simulink model "starmac_system_embedded_test"  (Simulink 7.1)
settings: Solver=ode23  StartTime=0.0  StopTime=80  FixedStep=.001  MaxStep=.01  RelTol=1e-4
libraries: aero_sim_lib x7, control_design_lib x6, simulink x4
(part 1 of 2)
settings Model: Creator=Administrator  LastModifiedBy=jporter

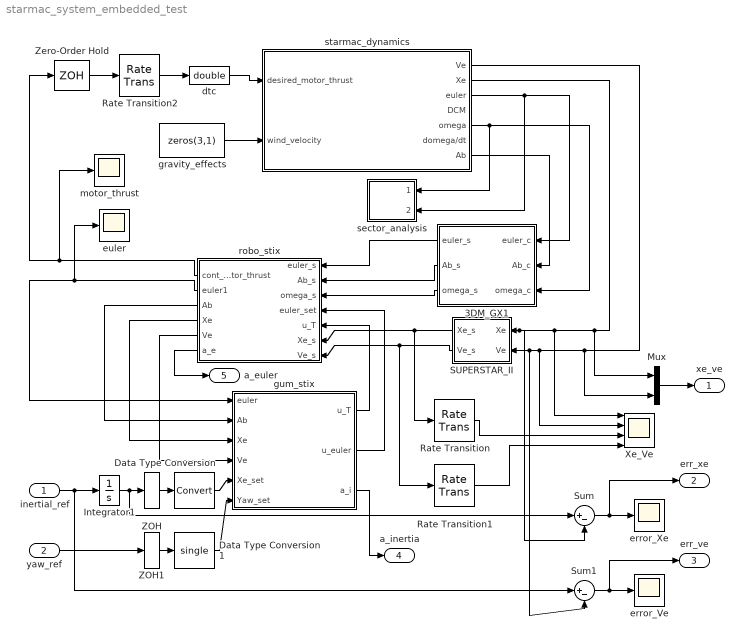
== system starmac_system_embedded_test ==
  inertial_ref : Inport  OutDataType=sfix(16)  OutScaling=2^0
  yaw_ref : Inport  Port=2  OutDataType=sfix(16)  OutScaling=2^0
  3DM_GX1 : Subsystem  Orientation=left  mask{a_g_s=7000, g_max=5, g_g_s=8500, omega_max=300, Ts=.02}
      mask prompts: a_g_s "AccelGainScale:"; g_max "Max G (1 G = 9.81 m/s^2):"; g_g_s "GyroGainScale:"; omega_max "Mav Angular Velocity (deg/sec):"; Ts "Sample Rate (seconds):"
  Data Type Conversion : DataTypeConversion  OutDataType=sfix(16)  OutScaling=2^0
  Data Type Conversion1 : DataTypeConversion  OutDataTypeMode=single  OutDataType=sfix(16)  OutScaling=2^0  OutDataTypeStr=single
  Integrator1 : Integrator
  Mux : Mux  Inputs=2
  Rate Transition : RateTransition
  Rate Transition1 : RateTransition
  Rate Transition2 : RateTransition
  SUPERSTAR_II : Subsystem  Orientation=left  mask{Ts=.02}
      mask prompts: Ts "Sample Rate (seconds):"
  Sum : Sum  Inputs=|+-  OutDataType=sfix(16)  OutScaling=2^0
  Sum1 : Sum  Inputs=|+-  OutDataType=sfix(16)  OutScaling=2^0
  Xe_Ve : Scope  NumInputPorts=4
      settings: YMin=-15~-6~-15~-6  YMax=15~5~15~5  Decimation=20
  ZOH : ZeroOrderHold  SampleTime=.02
  ZOH1 : ZeroOrderHold  SampleTime=.02
  Zero-Order Hold : ZeroOrderHold  SampleTime=.02
  dtc : DataTypeConversion  OutDataTypeMode=double  OutDataType=sfix(16)  OutScaling=2^0  OutDataTypeStr=double
  error_Ve : Scope
      settings: YMin=-4  SaveName=ScopeData14  Decimation=10
  error_Xe : Scope
      settings: YMin=-4  SaveName=ScopeData4  Decimation=10
  euler : Scope
      settings: TimeRange=60  YMin=-0.05  YMax=0.009999999999999995
  gravity_effects : Constant  Value=zeros(3,1)  OutDataTypeMode=double  OutDataType=sfix(16)  OutScaling=2^0  OutDataTypeStr=double
  gum_stix : Subsystem
  motor_thrust : Scope
      settings: YMin=2.5  YMax=10  SaveName=ScopeData3
  robo_stix : Subsystem  Orientation=left
  sector_analysis : Subsystem  Orientation=left
  starmac_dynamics : Subsystem  AncestorBlock=aero_sim_lib/starmac_dynamics  mask{M=1.8263, tau_motor=0.1, b=0.1, select_sub=Select Subsystem}
      mask prompts: M "UAV Mass (kg) [M]:"; tau_motor "Motor Time constant (s)[tau_motor]:"; b "Viscus Drag Coef. (N-s/m)[b]:"; select_sub "Select a model Subsystem:"
      mask StyleString: edit,edit,edit,popup(Select Subsystem|M:starmac_motor_dynamics|B:starmac_blade_flapping_effects|6:6DOF_Euler_Angles)
      mask CallbackString:
      | |||gcb_d=gcb;
      | mask_str = get_param(gcb_d, 'MaskValues');
      | if strcmp(mask_str{4}(1),'M')
      |     open_system([gcb_d '/starmac_motor_dynamics'],'mask');
      | elseif strcmp(mask_str{4}(1),'B')
      |     open_system([gcb_d '/starmac_blade_flapping_effects'],'mask');
      | elseif strcmp(mask_str{4}(1),'6')
      |     open_system([gcb_d '/6DOF_Euler_Angles'],'mask');
      | else
      |     return
      | end
      | set_param(gcb_d,'select_sub','Select Subsystem');
  xe_ve : Outport
  err_xe : Outport  Port=2
  err_ve : Outport  Port=3
  a_inertia : Outport  Port=4
  a_euler : Outport  Port=5
  wires:
  robo_stix/1(cont_motor_thrust) -> Zero-Order Hold/1, motor_thrust/1
  starmac_dynamics/3(euler) -> 3DM_GX1/1(euler_c), sector_analysis/2(out(eta))
  starmac_dynamics/7(Ab) -> 3DM_GX1/2(Ab_c)
  3DM_GX1/1(euler_s) -> robo_stix/1(euler_s)
  3DM_GX1/2(Ab_s) -> robo_stix/2(Ab_s)
  3DM_GX1/3(omega_s) -> robo_stix/3(omega_s)
  robo_stix/2(euler1) -> euler/1, gum_stix/1(euler)
  SUPERSTAR_II/1(Xe_s) -> Rate Transition/1, robo_stix/6(Xe_s)
  SUPERSTAR_II/2(Ve_s) -> Rate Transition1/1, robo_stix/7(Ve_s)
  starmac_dynamics/2(Xe) -> Xe_Ve/1, SUPERSTAR_II/1(Xe), Sum/2, Mux/1
  starmac_dynamics/1(Ve) -> Xe_Ve/2, SUPERSTAR_II/2(Ve), Sum1/2, Mux/2
  inertial_ref/1 -> Integrator1/1, Sum1/1
  gravity_effects/1 -> starmac_dynamics/2(wind_velocity)
  Sum/1 -> error_Xe/1, err_xe/1
  Rate Transition/1 -> Xe_Ve/3
  Rate Transition1/1 -> Xe_Ve/4
  gum_stix/1(u_T) -> robo_stix/5(u_T)
  gum_stix/2(u_euler) -> robo_stix/4(euler_set)
  Data Type Conversion/1 -> gum_stix/5(Xe_set)
  dtc/1 -> starmac_dynamics/1(desired_motor_thrust)
  starmac_dynamics/5(omega) -> 3DM_GX1/3(omega_c), sector_analysis/1(in(omega))
  Zero-Order Hold/1 -> Rate Transition2/1
  Rate Transition2/1 -> dtc/1
  robo_stix/3(Ab) -> gum_stix/2(Ab)
  robo_stix/4(Xe) -> gum_stix/3(Xe)
  robo_stix/5(Ve) -> gum_stix/4(Ve)
  Integrator1/1 -> ZOH/1, Sum/1
  ZOH/1 -> Data Type Conversion/1
  ZOH1/1 -> Data Type Conversion1/1
  yaw_ref/1 -> ZOH1/1
  Data Type Conversion1/1 -> gum_stix/6(Yaw_set)
  Mux/1 -> xe_ve/1
  Sum1/1 -> error_Ve/1, err_ve/1
  gum_stix/3(a_i) -> a_inertia/1
  robo_stix/6(a_e) -> a_euler/1

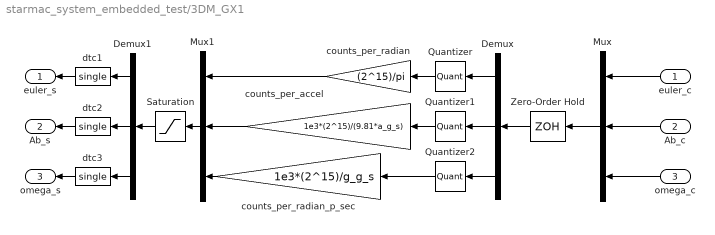
== system starmac_system_embedded_test/3DM_GX1 ==
  euler_c : Inport  Orientation=left
  Ab_c : Inport  Orientation=left  Port=2
  omega_c : Inport  Orientation=left  Port=3
  Demux : Demux  Orientation=left  Outputs=[3 3 3]
  Demux1 : Demux  Orientation=left  Outputs=[3 3 3]
  Mux : Mux  Orientation=left  Inputs=[3 3 3]
  Mux1 : Mux  Orientation=left  Inputs=3
  Quantizer : Quantizer  Orientation=left  QuantizationInterval=pi/(2^15)*ones(3,1)
  Quantizer1 : Quantizer  Orientation=left  QuantizationInterval=g_max*9.81/(2^15)*ones(3,1)
  Quantizer2 : Quantizer  Orientation=left  QuantizationInterval=(pi*omega_max/180)/(2^15)*ones(3,1)
  Saturation : Saturate  Orientation=left  UpperLimit=((2^15)-1)*ones(3*3,1)  LowerLimit=-(2^15)*ones(3*3,1)  OutDataType=sfix(16)  OutScaling=2^0
  Zero-Order Hold : ZeroOrderHold  Orientation=left  SampleTime=Ts
  counts_per_accel : Gain  Orientation=left  Gain=1e3*(2^15)/(9.81*a_g_s)  ParameterDataType=sfix(16)  ParameterScaling=2^0  OutDataType=sfix(16)  OutScaling=2^0
  counts_per_radian : Gain  Orientation=left  Gain=(2^15)/pi  ParameterDataType=sfix(16)  ParameterScaling=2^0  OutDataType=sfix(16)  OutScaling=2^0
  counts_per_radian_p_sec : Gain  Orientation=left  Gain=1e3*(2^15)/g_g_s  ParameterDataType=sfix(16)  ParameterScaling=2^0  OutDataType=sfix(16)  OutScaling=2^0
  dtc1 : DataTypeConversion  Orientation=left  OutDataTypeMode=single  OutDataType=sfix(16)  OutScaling=2^0  OutDataTypeStr=single
  dtc2 : DataTypeConversion  Orientation=left  OutDataTypeMode=single  OutDataType=sfix(16)  OutScaling=2^0  OutDataTypeStr=single
  dtc3 : DataTypeConversion  Orientation=left  OutDataTypeMode=single  OutDataType=sfix(16)  OutScaling=2^0  OutDataTypeStr=single
  euler_s : Outport  Orientation=left
  Ab_s : Outport  Orientation=left  Port=2
  omega_s : Outport  Orientation=left  Port=3
  wires:
  Mux/1 -> Zero-Order Hold/1
  euler_c/1 -> Mux/1
  Ab_c/1 -> Mux/2
  omega_c/1 -> Mux/3
  Zero-Order Hold/1 -> Demux/1
  Demux/1 -> Quantizer/1
  Demux/2 -> Quantizer1/1
  Quantizer/1 -> counts_per_radian/1
  Quantizer1/1 -> counts_per_accel/1
  counts_per_accel/1 -> Mux1/2
  counts_per_radian/1 -> Mux1/1
  Demux/3 -> Quantizer2/1
  counts_per_radian_p_sec/1 -> Mux1/3
  Quantizer2/1 -> counts_per_radian_p_sec/1
  Mux1/1 -> Saturation/1
  Saturation/1 -> Demux1/1
  Demux1/1 -> dtc1/1
  Demux1/2 -> dtc2/1
  Demux1/3 -> dtc3/1
  dtc1/1 -> euler_s/1
  dtc2/1 -> Ab_s/1
  dtc3/1 -> omega_s/1

== system starmac_system_embedded_test/SUPERSTAR_II ==
  Xe : Inport  Orientation=left
  Ve : Inport  Orientation=left  Port=2
  Demux : Demux  Orientation=left  Outputs=[3 3]
  Mux : Mux  Orientation=left  Inputs=[3 3]
  Rate Transition : RateTransition  Orientation=left
  ZOH : ZeroOrderHold  Orientation=left  SampleTime=Ts
  dtc1 : DataTypeConversion  Orientation=left  OutDataTypeMode=single  OutDataType=sfix(16)  OutScaling=2^0  OutDataTypeStr=single
  dtc2 : DataTypeConversion  Orientation=left  OutDataTypeMode=single  OutDataType=sfix(16)  OutScaling=2^0  OutDataTypeStr=single
  Xe_s : Outport  Orientation=left
  Ve_s : Outport  Orientation=left  Port=2
  wires:
  ZOH/1 -> Rate Transition/1
  Ve/1 -> Mux/2
  Xe/1 -> Mux/1
  Mux/1 -> ZOH/1
  Demux/1 -> dtc1/1
  Demux/2 -> dtc2/1
  dtc1/1 -> Xe_s/1
  dtc2/1 -> Ve_s/1
  Rate Transition/1 -> Demux/1

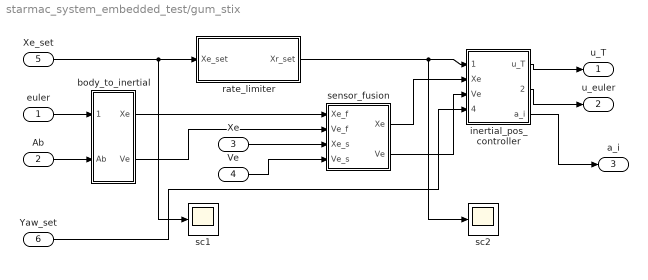
== system starmac_system_embedded_test/gum_stix ==
  euler : Inport  PortDimensions=[3]  DataType=single  OutDataTypeStr=single
  Ab : Inport  Port=2  PortDimensions=[3]  DataType=single  OutDataTypeStr=single
  Xe : Inport  Port=3  PortDimensions=[3]  DataType=single  OutDataTypeStr=single
  Ve : Inport  Port=4  PortDimensions=[3]  DataType=single  OutDataTypeStr=single
  Xe_set : Inport  Port=5  PortDimensions=[3]  DataType=single  OutDataTypeStr=single
  Yaw_set : Inport  Port=6  PortDimensions=[1]  DataType=single  OutDataTypeStr=single
  body_to_inertial : Subsystem
  inertial_pos_controller : Subsystem
  rate_limiter : Subsystem  mask{wn=2*pi, zeta=0.9, Vmax=2, Tsamp=0.02}
      mask prompts: wn "omega_n"; Vmax "Max velocity"; Tsamp "Sample time"
      mask init:
      | Fsys = tf([wn^2],[1,2*zeta*wn,wn^2]);
      | Fd = c2d( Fsys, Tsamp, 'zoh' );
      | FS = ss( Fd );
      | Add = FS.a;
      | Bdd = FS.b;
      | Cdd = FS.c;
      | Ddd = FS.d;
      | %Add = blkdiag(FS.a, FS.a, FS.a );
      | %Bdd = blkdiag(FS.b, FS.b, FS.b );
      | %Cdd = blkdiag(FS.c, FS.c, FS.c );
      | %Ddd = blkdiag(FS.d, FS.d, FS.d );
      | %Sdd = ss( Add, Bdd, Cdd, Ddd, Tsamp );
  sc1 : Scope
      settings: YMin=-7.5  YMax=22.5  SaveName=ScopeData8  Decimation=10
  sc2 : Scope
      settings: YMin=-2  YMax=2  SaveName=ScopeData9  Decimation=10
  sensor_fusion : Subsystem
  u_T : Outport  PortDimensions=[1]  DataType=single  OutDataTypeStr=single
  u_euler : Outport  Port=2  PortDimensions=[3]  DataType=single  OutDataTypeStr=single
  a_i : Outport  Port=3
  wires:
  Xe_set/1 -> rate_limiter/1(Xe_set), sc1/1
  inertial_pos_controller/1(u_T) -> u_T/1
  inertial_pos_controller/2(u_euler) -> u_euler/1
  euler/1 -> body_to_inertial/1(euler)
  Ab/1 -> body_to_inertial/2(Ab)
  sensor_fusion/1(Xe) -> inertial_pos_controller/2(Xe)
  sensor_fusion/2(Ve) -> inertial_pos_controller/3(Ve)
  body_to_inertial/1(Xe) -> sensor_fusion/1(Xe_f)
  body_to_inertial/2(Ve) -> sensor_fusion/2(Ve_f)
  Xe/1 -> sensor_fusion/3(Xe_s)
  Ve/1 -> sensor_fusion/4(Ve_s)
  rate_limiter/1(Xr_set) -> inertial_pos_controller/1(Xe_set), sc2/1
  Yaw_set/1 -> inertial_pos_controller/4(Yaw_set)
  inertial_pos_controller/3(a_i) -> a_i/1

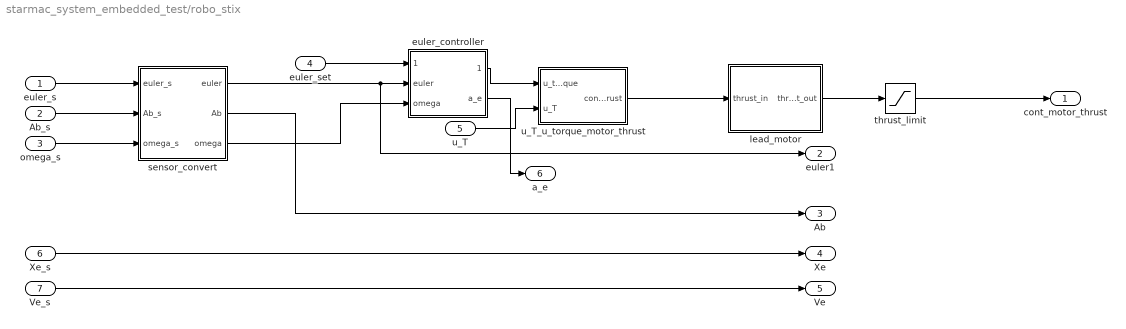
== system starmac_system_embedded_test/robo_stix ==
  euler_s : Inport  PortDimensions=[3]  DataType=single  OutDataTypeStr=single
  Ab_s : Inport  Port=2  PortDimensions=[3]  DataType=single  OutDataTypeStr=single
  omega_s : Inport  Port=3  PortDimensions=[3]  DataType=single  OutDataTypeStr=single
  euler_set : Inport  Port=4  PortDimensions=[3]  DataType=single  OutDataTypeStr=single
  u_T : Inport  Port=5  PortDimensions=[1]  DataType=single  OutDataTypeStr=single
  Xe_s : Inport  Port=6  PortDimensions=[3]  DataType=single  OutDataTypeStr=single
  Ve_s : Inport  Port=7  PortDimensions=[3]  DataType=single  OutDataTypeStr=single
  euler_controller : Subsystem  mask{K=1, K_e=7.5, K_o=.65}
      mask prompts: K "Loop Gain [K]:"; K_e "Euler Gain [K_e]:"; K_o "Omega Gain [K_o]:"
  lead_motor : Subsystem  mask{tau_motor=.1, t_s=.020}
      mask init:
      | a=1/tau_motor;
      | b=pi/t_s;
      | T=t_s;
      | num1=b*(1-exp(-b*T))+a*(b*T-1+exp(-b*T));
      | num2=-b*(1-exp(-b*T))+a*(1-exp(-b*T)-b*T*exp(-b*T));
      | den1=a*b;
      | den2=-a*b*exp(-b*T);
      | num=[num1 num2];
      | den=[den1 den2];
      | Hz=tf(num,den,T);
      | [y,t]=step(Hz);
      | k_ss=(1/y(length(y)));
      | num=k_ss*num;
      | lead_a_1=single(-den(2)/den(1))
      | lead_b_1=single(num(2)/den(1))
      | lead_b_2=single(num(1)/den(1))
      | %Hz=k_ss*Hz
      | %bode(Hz);
  sensor_convert : Subsystem  mask{a_g_s=7000, g_g_s=8500}
      mask prompts: a_g_s "AccelGainScale[a_g_s]:"; g_g_s "GyroGainScale[g_g_s]:"
  thrust_limit : Saturate  UpperLimit=10*ones(4,1)  LowerLimit=0*ones(4,1)  OutDataTypeMode=single  OutDataType=sfix(16)  OutScaling=2^0  OutDataTypeStr=single
  u_T_u_torque_motor_thrust : Subsystem  mask{dx=.3048, K_torque=.47}
      mask prompts: dx "X distance of motor from CG [dx](meters):"; K_torque "Ktorque [K_torque]:"
      mask init:
      | M=[0 -dx 0 dx;
      |    dx 0 -dx 0;
      |    -K_torque K_torque -K_torque K_torque;
      |    1 1 1 1];
      | Mi=inv(M);
  cont_motor_thrust : Outport
  euler1 : Outport  Port=2
  Ab : Outport  Port=3
  Xe : Outport  Port=4
  Ve : Outport  Port=5
  a_e : Outport  Port=6
  wires:
  euler_s/1 -> sensor_convert/1(euler_s)
  Ab_s/1 -> sensor_convert/2(Ab_s)
  omega_s/1 -> sensor_convert/3(omega_s)
  sensor_convert/1(euler) -> euler_controller/2(euler), euler1/1
  euler_set/1 -> euler_controller/1(euler_set)
  sensor_convert/3(omega) -> euler_controller/3(omega)
  u_T/1 -> u_T_u_torque_motor_thrust/2(u_T)
  euler_controller/1(u_torque) -> u_T_u_torque_motor_thrust/1(u_torque)
  sensor_convert/2(Ab) -> Ab/1
  Ve_s/1 -> Ve/1
  thrust_limit/1 -> cont_motor_thrust/1
  Xe_s/1 -> Xe/1
  u_T_u_torque_motor_thrust/1(cont_motor_thrust) -> lead_motor/1(thrust_in)
  lead_motor/1(thrust_out) -> thrust_limit/1
  euler_controller/2(a_e) -> a_e/1

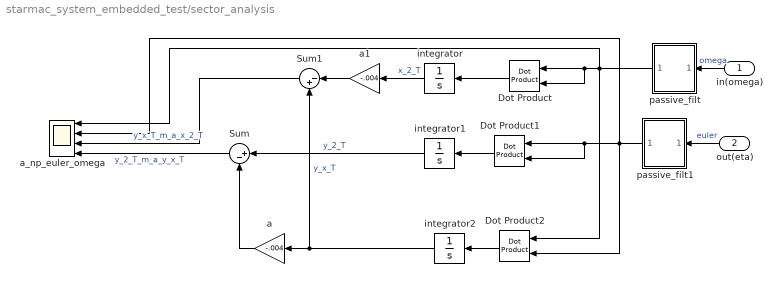
== system starmac_system_embedded_test/sector_analysis ==
  in(omega) : Inport  Orientation=left
  out(eta) : Inport  Orientation=left  Port=2
  Dot Product : simulink/Math Operations/Dot Product  Orientation=left  InputSameDT=on  OutDataType=sfix(16)  OutScaling=2^-10  DoSatur=off
  Dot Product1 : simulink/Math Operations/Dot Product  Orientation=left  InputSameDT=on  OutDataType=sfix(16)  OutScaling=2^-10  DoSatur=off
  Dot Product2 : simulink/Math Operations/Dot Product  Orientation=left  InputSameDT=on  OutDataType=sfix(16)  OutScaling=2^-10  DoSatur=off
  Sum : Sum  Orientation=left  Inputs=|+-  OutDataType=sfix(16)  OutScaling=2^0
  Sum1 : Sum  Orientation=left  Inputs=|-+  OutDataType=sfix(16)  OutScaling=2^0
  a : Gain  Orientation=left  Gain=-.004  ParameterDataType=sfix(16)  ParameterScaling=2^0  OutDataType=sfix(16)  OutScaling=2^0
  a1 : Gain  Orientation=left  Gain=-.004  ParameterDataType=sfix(16)  ParameterScaling=2^0  OutDataType=sfix(16)  OutScaling=2^0
  a_np_euler_omega : Scope  NumInputPorts=4
      settings: YMin=-0.3~-0.3~-3.46945e-018~5.5  YMax=0.3~0.4~0.13~8.5  SaveName=ScopeData6  Decimation=2
  integrator : Integrator  Orientation=left
  integrator1 : Integrator  Orientation=left
  integrator2 : Integrator  Orientation=left
  passive_filt : Subsystem  Orientation=left  mask{omega_n=10*2*pi, zeta=1}
  passive_filt1 : Subsystem  Orientation=left  mask{omega_n=10*2*pi, zeta=1}
  wires:
  Dot Product/1 -> integrator/1
  Dot Product1/1 -> integrator1/1
  integrator1/1 -> Sum/1  "y_2_T"
  out(eta)/1 -> passive_filt1/1(In1)  "euler"
  in(omega)/1 -> passive_filt/1(In1)  "omega"
  Dot Product2/1 -> integrator2/1
  integrator2/1 -> a/1, Sum1/2  "y_x_T"
  integrator/1 -> a1/1  "x_2_T"
  a/1 -> Sum/2
  a1/1 -> Sum1/1
  Sum/1 -> a_np_euler_omega/4  "y_2_T_m_a_y_x_T"
  Sum1/1 -> a_np_euler_omega/3  "y_x_T_m_a_x_2_T"
  passive_filt/1(Out1) -> Dot Product/1, Dot Product/2, Dot Product2/1, a_np_euler_omega/1
  passive_filt1/1(Out1) -> Dot Product1/1, Dot Product1/2, Dot Product2/2, a_np_euler_omega/2

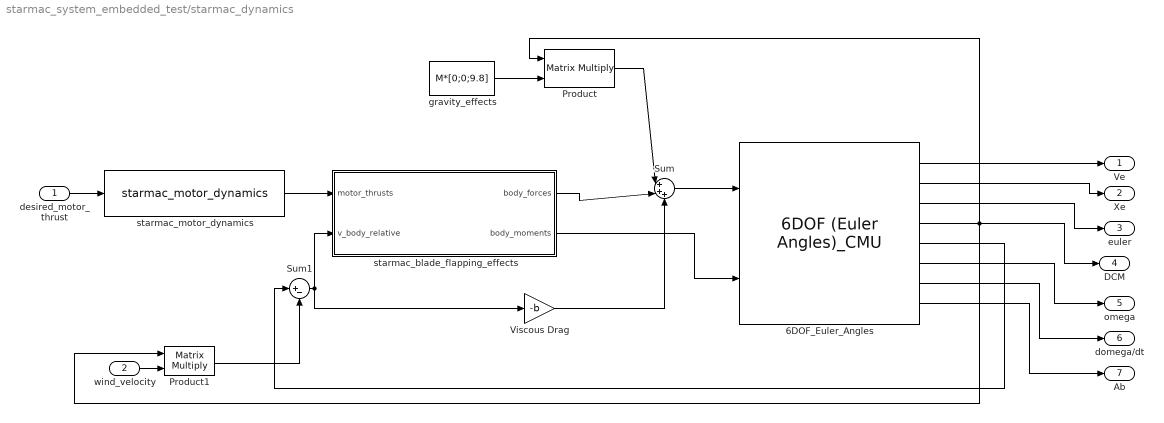
== system starmac_system_embedded_test/starmac_dynamics ==
  desired_motor_thrust : Inport  OutDataType=sfix(16)  OutScaling=2^0
  wind_velocity : Inport  Port=2  OutDataType=sfix(16)  OutScaling=2^0
  6DOF_Euler_Angles : aero_sim_lib/6DOF (Euler Angles)_CMU  SystemSampleTime=-1  XYZe_0=[0.1;0.2;0]  Vb_0=[0;0;0]  euler_0=[0;0;0]  omega_0=[0;0;0]  M=M  I=diag([0.02759 0.02771 0.04806])
  Product : Product  Multiplication=Matrix(*)  OutDataType=sfix(16)  OutScaling=2^0  RndMeth=Zero
  Product1 : Product  Multiplication=Matrix(*)  OutDataType=sfix(16)  OutScaling=2^0  RndMeth=Zero
  Sum : Sum  Inputs=|+++  OutDataType=sfix(16)  OutScaling=2^0
  Sum1 : Sum  Inputs=|+-  OutDataType=sfix(16)  OutScaling=2^0
  Viscous Drag : Gain  Gain=-b  ParameterDataType=sfix(16)  ParameterScaling=2^0  OutDataType=sfix(16)  OutScaling=2^0
  gravity_effects : Constant  Value=M*[0;0;9.8]  OutDataType=sfix(16)  OutScaling=2^0
  starmac_blade_flapping_effects : Subsystem  AncestorBlock=aero_sim_lib/starmac_blade_flapping_effects  mask{select_sub=Select Subsystem}
      mask prompts: select_sub "Select Subsystem:"
      mask help:
      | Allows user to set parameters of various subsystems
      | within the Blade Flapping Effects Model
      mask Help:
      | Select a Subsystem To Set Various
      | Sub System Parameters
      mask StyleString: popup(Select Subsystem|V:starmac_vertical_effect_dynamics|B:starmac_body_moments|F:starmac_flapping_dynamics)
      mask CallbackString:
      | gcb_c=gcb;
      | mask_str = get_param(gcb_c, 'MaskValues');
      | if strcmp(mask_str{1}(1),'V')
      |     open_system([gcb_c '/starmac_vertical_effect_dynamics'],'mask');
      | elseif strcmp(mask_str{1}(1),'B')
      |     open_system([gcb_c '/starmac_body_moments'],'mask');
      | elseif strcmp(mask_str{1}(1),'F')
      |     open_system([gcb_c '/starmac_flapping_dynamics'],'mask');
      | else
      |     return
      | end
      | set_param(gcb_c,'select_sub','Select Subsystem');
  starmac_motor_dynamics : aero_sim_lib/starmac_motor_dynamics  SystemSampleTime=-1  tau_motor=tau_motor  T_nom=M*9.8/4  thrust_max=9.8  thrust_min=0  motor_lag_enable=on  motor_variance=(.05*9.8/4)^2  Ts=1/76
  Ve : Outport  OutDataType=sfix(16)  OutScaling=2^0
  Xe : Outport  Port=2  OutDataType=sfix(16)  OutScaling=2^0
  euler : Outport  Port=3  OutDataType=sfix(16)  OutScaling=2^0
  DCM : Outport  Port=4  OutDataType=sfix(16)  OutScaling=2^0
  omega : Outport  Port=5  OutDataType=sfix(16)  OutScaling=2^0
  domega/dt : Outport  Port=6  OutDataType=sfix(16)  OutScaling=2^0
  Ab : Outport  Port=7  OutDataType=sfix(16)  OutScaling=2^0
  wires:
  6DOF_Euler_Angles/8 -> Ab/1
  6DOF_Euler_Angles/7 -> domega/dt/1
  6DOF_Euler_Angles/6 -> omega/1
  6DOF_Euler_Angles/3 -> euler/1
  6DOF_Euler_Angles/2 -> Xe/1
  6DOF_Euler_Angles/1 -> Ve/1
  starmac_motor_dynamics/1 -> starmac_blade_flapping_effects/1(motor_thrusts)
  Product/1 -> Sum/1
  Sum/1 -> 6DOF_Euler_Angles/1
  6DOF_Euler_Angles/4 -> DCM/1, Product/1, Product1/1
  gravity_effects/1 -> Product/2
  Sum1/1 -> starmac_blade_flapping_effects/2(v_body_relative), Viscous Drag/1
  Product1/1 -> Sum1/2
  6DOF_Euler_Angles/5 -> Sum1/1
  Viscous Drag/1 -> Sum/3
  starmac_blade_flapping_effects/2(body_moments) -> 6DOF_Euler_Angles/2
  starmac_blade_flapping_effects/1(body_forces) -> Sum/2
  desired_motor_thrust/1 -> starmac_motor_dynamics/1
  wind_velocity/1 -> Product1/2

== system starmac_system_embedded_test/gum_stix/body_to_inertial ==
  euler : Inport
  Ab : Inport  Port=2
  Ab_to_Ae : Stateflow chart
  inertial_vel_and pos_est : Subsystem  mask{Ts=.02}
      mask prompts: Ts "Sample Time [Ts] (seconds):"
  Xe : Outport
  Ve : Outport  Port=2
  wires:
  euler/1 -> Ab_to_Ae/1(euler)
  Ab/1 -> Ab_to_Ae/2(Ab)
  Ab_to_Ae/1(Ae) -> inertial_vel_and pos_est/1(Ab)
  inertial_vel_and pos_est/1(Vb) -> Ve/1
  inertial_vel_and pos_est/2(Xb) -> Xe/1

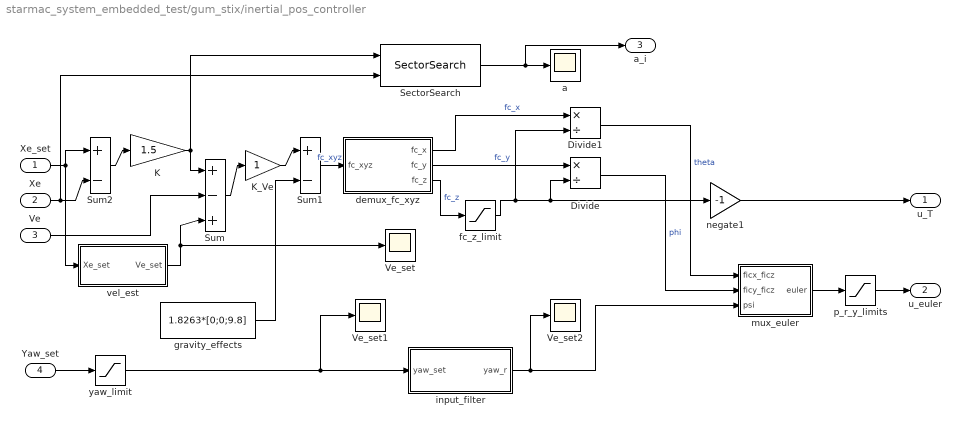
== system starmac_system_embedded_test/gum_stix/inertial_pos_controller ==
  Xe_set : Inport
  Xe : Inport  Port=2
  Ve : Inport  Port=3
  Yaw_set : Inport  Port=4
  Divide : Product  Inputs=*/  OutDataTypeMode=single  OutDataType=sfix(16)  OutScaling=2^-10  OutDataTypeStr=single
  Divide1 : Product  Inputs=*/  OutDataTypeMode=single  OutDataType=sfix(16)  OutScaling=2^-10  OutDataTypeStr=single
  K : Gain  Gain=1.5  ParameterDataType=sfix(16)  ParameterScaling=2^0  OutDataTypeMode=single  OutDataType=sfix(16)  OutScaling=2^0  OutDataTypeStr=single
  K_Ve : Gain  ParameterDataTypeMode=single  ParameterDataType=sfix(16)  ParameterScaling=2^0  ParamDataTypeStr=single  OutDataTypeMode=single  OutDataType=sfix(16)  OutScaling=2^0  OutDataTypeStr=single
  SectorSearch : control_design_lib/SectorSearch  SystemSampleTime=-1
  Sum : Sum  Inputs=|+-+  AccumDataTypeStr=single  OutDataTypeMode=single  OutDataType=sfix(16)  OutScaling=2^0  OutDataTypeStr=single
  Sum1 : Sum  Inputs=|+-  AccumDataTypeStr=single  OutDataTypeMode=single  OutDataType=sfix(16)  OutScaling=2^0  OutDataTypeStr=single
  Sum2 : Sum  Inputs=|+-  AccumDataTypeStr=single  OutDataTypeMode=single  OutDataType=sfix(16)  OutScaling=2^0  OutDataTypeStr=single
  Ve_set : Scope
      settings: TimeRange=60  SaveName=ScopeData2  Decimation=10
  Ve_set1 : Scope
      settings: TimeRange=60  SaveName=ScopeData10  Decimation=10
  Ve_set2 : Scope
      settings: TimeRange=60  SaveName=ScopeData11  Decimation=10
  a : Scope
      settings: YMin=-2  YMax=2  SaveName=ScopeData13  Decimation=10
  demux_fc_xyz : Stateflow chart
  fc_z_limit : Saturate  UpperLimit=-(1/8)*9.81  LowerLimit=-4*9.81  OutDataTypeMode=single  OutDataType=sfix(16)  OutScaling=2^0  OutDataTypeStr=single
  gravity_effects : Constant  Value=1.8263*[0;0;9.8]  OutDataTypeMode=single  OutDataType=sfix(16)  OutScaling=2^0  OutDataTypeStr=single
  input_filter : Subsystem  mask{wn=1, zeta=0.9, Tsamp=0.02}
      mask prompts: wn "omega_n"; Tsamp "Sample time"
      mask init: same as starmac_system_embedded_test/gum_stix/rate_limiter
  mux_euler : Stateflow chart
  negate1 : Gain  Gain=-1  ParameterDataType=sfix(16)  ParameterScaling=2^0  OutDataTypeMode=single  OutDataType=sfix(16)  OutScaling=2^0  OutDataTypeStr=single
  p_r_y_limits : Saturate  UpperLimit=(pi/4)*ones(1,3)  LowerLimit=-(pi/4)*ones(1,3)  OutDataTypeMode=single  OutDataType=sfix(16)  OutScaling=2^0  OutDataTypeStr=single
  vel_est : Subsystem  mask{tau_f=.02/pi, T=.02}
      mask prompts: T "sample rate"
      mask init:
      | b=1/tau_f;
      | num1=(1-exp(-b*T));
      | num2=-num1;
      | den1=1;
      | den2=-exp(-b*T);
      | num=(1/T)*[num1 num2];
      | den=[den1 den2];
      | vel_est_a_1=single(-den(2)/den(1))
      | vel_est_b_1=single(num(2)/den(1))
      | vel_est_b_2=single(num(1)/den(1))
      | %Hz=tf(num,den,T);
      | %bode(Hz);
      | %hold on;
      | %bode(tf([1 0],[tau_f 1]));
  yaw_limit : Saturate  UpperLimit=pi  LowerLimit=-pi  OutDataTypeMode=single  OutDataType=sfix(16)  OutScaling=2^0  OutDataTypeStr=single
  u_T : Outport
  u_euler : Outport  Port=2
  a_i : Outport  Port=3
  wires:
  fc_z_limit/1 -> Divide1/2, Divide/2, negate1/1
  Xe_set/1 -> Sum2/1, vel_est/1(Xe_set)
  negate1/1 -> u_T/1
  p_r_y_limits/1 -> u_euler/1
  demux_fc_xyz/1(fc_x) -> Divide1/1  "fc_x"
  demux_fc_xyz/3(fc_z) -> fc_z_limit/1  "fc_z"
  mux_euler/1(euler) -> p_r_y_limits/1
  Sum1/1 -> demux_fc_xyz/1(fc_xyz)  "fc_xyz"
  gravity_effects/1 -> Sum1/2
  Sum/1 -> K_Ve/1
  Xe/1 -> Sum2/2, SectorSearch/2
  Sum2/1 -> K/1
  K/1 -> Sum/1, SectorSearch/1
  demux_fc_xyz/2(fc_y) -> Divide/1  "fc_y"
  K_Ve/1 -> Sum1/1
  Ve/1 -> Sum/2
  vel_est/1(Ve_set) -> Sum/3, Ve_set/1
  Divide1/1 -> mux_euler/1(ficx_ficz)  "theta"
  Divide/1 -> mux_euler/2(ficy_ficz)  "phi"
  Yaw_set/1 -> yaw_limit/1
  yaw_limit/1 -> input_filter/1(yaw_set), Ve_set1/1
  input_filter/1(yaw_r) -> mux_euler/3(psi), Ve_set2/1
  SectorSearch/1 -> a/1, a_i/1

== system starmac_system_embedded_test/gum_stix/rate_limiter ==
  Xe_set : Inport  OutDataType=sfix(16)  OutScaling=2^0
  Constant : Constant  Value=Tsamp  OutDataTypeMode=single  OutDataType=sfix(16)  OutScaling=2^0  OutDataTypeStr=single
  Constant1 : Constant  Value=Vmax  OutDataTypeMode=single  OutDataType=sfix(16)  OutScaling=2^0  OutDataTypeStr=single
  Demux : Demux  Outputs=3
  Embedded MATLAB Function : Stateflow chart
  LinDiscSS : control_design_lib/LinDiscSS  SystemSampleTime=-1  Add=Add  Bdd=Bdd  Cdd=Cdd  Ddd=Ddd  x0=0  Tsamp=Tsamp
  LinDiscSS1 : control_design_lib/LinDiscSS  SystemSampleTime=-1  Add=Add  Bdd=Bdd  Cdd=Cdd  Ddd=Ddd  x0=0  Tsamp=Tsamp
  LinDiscSS2 : control_design_lib/LinDiscSS  SystemSampleTime=-1  Add=Add  Bdd=Bdd  Cdd=Cdd  Ddd=Ddd  x0=0  Tsamp=Tsamp
  Mux : Mux  Inputs=3
  Unit Delay : UnitDelay  Orientation=left  SampleTime=-1
  Xr_set : Outport  OutDataType=sfix(16)  OutScaling=2^0
  wires:
  Xe_set/1 -> Demux/1
  Mux/1 -> Embedded MATLAB Function/1(Xd)
  Embedded MATLAB Function/1(Xr) -> Xr_set/1, Unit Delay/1
  Unit Delay/1 -> Embedded MATLAB Function/2(Xd_prev)
  Constant/1 -> Embedded MATLAB Function/3(Tsamp)
  Constant1/1 -> Embedded MATLAB Function/4(Vmax)
  Demux/1 -> LinDiscSS/1
  LinDiscSS/1 -> Mux/1
  Demux/2 -> LinDiscSS1/1
  LinDiscSS1/1 -> Mux/2
  Demux/3 -> LinDiscSS2/1
  LinDiscSS2/1 -> Mux/3

== system starmac_system_embedded_test/gum_stix/sensor_fusion ==
  Xe_f : Inport
  Ve_f : Inport  Port=2
  Xe_s : Inport  Port=3
  Ve_s : Inport  Port=4
  Sum : Sum  Inputs=|+-  OutDataTypeMode=single  OutDataType=sfix(16)  OutScaling=2^0  OutDataTypeStr=single
  Sum1 : Sum  Inputs=|+-  OutDataTypeMode=single  OutDataType=sfix(16)  OutScaling=2^0  OutDataTypeStr=single
  delays : Subsystem  Orientation=left
  if_end : Subsystem
  if_end1 : Subsystem
  Xe : Outport
  Ve : Outport  Port=2
  wires:
  Xe_f/1 -> if_end/2(Xe_f), Sum/1
  delays/2(dX_1) -> if_end/3(dX_1p)
  Xe_s/1 -> if_end/1(Xe_s)
  delays/4(Xe_sh_1) -> if_end/4(Xe_sh_1p)
  Ve_f/1 -> if_end1/2(Ve_f), Sum1/1
  Ve_s/1 -> if_end1/1(Ve_s)
  delays/1(dV_1) -> if_end1/3(dV_1p)
  delays/3(Ve_sh_1) -> if_end1/4(Ve_sh_1p)
  if_end/2(dX_1) -> delays/2(dX), Sum/2
  if_end1/2(dV_1) -> delays/1(dV), Sum1/2
  if_end1/1(Ve_sh_1) -> delays/3(Ve_sh)
  if_end/1(Xe_sh_1) -> delays/4(Xe_sh)
  Sum/1 -> Xe/1
  Sum1/1 -> Ve/1

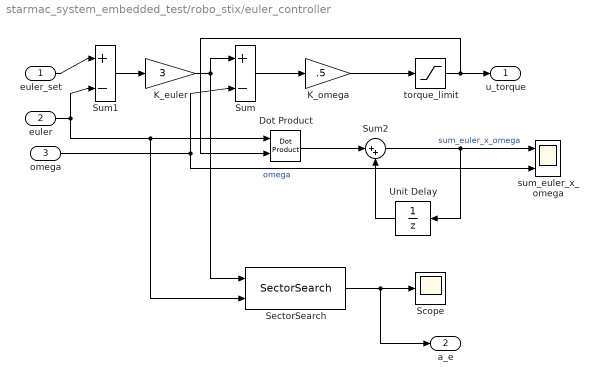
== system starmac_system_embedded_test/robo_stix/euler_controller ==
  euler_set : Inport
  euler : Inport  Port=2
  omega : Inport  Port=3
  Dot Product : simulink/Math Operations/Dot Product  InputSameDT=on  OutDataType=sfix(16)  OutScaling=2^-10  DoSatur=off
  K_euler : Gain  Gain=3  ParameterDataType=sfix(16)  ParameterScaling=2^0  OutDataType=sfix(16)  OutScaling=2^0
  K_omega : Gain  Gain=.5  ParameterDataType=sfix(16)  ParameterScaling=2^0  OutDataTypeMode=single  OutDataType=sfix(16)  OutScaling=2^0  OutDataTypeStr=single
  Scope : Scope
      settings: TimeRange=80  YMin=-1  YMax=1  SaveName=ScopeData12  MaxDataPoints=50000
  SectorSearch : control_design_lib/SectorSearch  SystemSampleTime=-1
  Sum : Sum  Inputs=|+-  AccumDataTypeStr=single  OutDataType=sfix(16)  OutScaling=2^0
  Sum1 : Sum  Inputs=|+-  AccumDataTypeStr=single  OutDataType=sfix(16)  OutScaling=2^0
  Sum2 : Sum  Inputs=|++  OutDataType=sfix(16)  OutScaling=2^0
  Unit Delay : UnitDelay  Orientation=left  SampleTime=-1
  sum_euler_x_omega : Scope  NumInputPorts=2
      settings: YMin=-0.5~-5  YMax=2~5  SaveName=ScopeData5  Decimation=20
  torque_limit : Saturate  UpperLimit=9.8*.3048*ones(3,1)  LowerLimit=-9.8*.3048*ones(3,1)  OutDataTypeMode=single  OutDataType=sfix(16)  OutScaling=2^0  OutDataTypeStr=single
  u_torque : Outport
  a_e : Outport  Port=2
  wires:
  Sum/1 -> K_omega/1
  euler_set/1 -> Sum1/1
  Sum1/1 -> K_euler/1
  euler/1 -> Sum1/2, Dot Product/1, SectorSearch/2
  K_euler/1 -> Sum/1, SectorSearch/1
  torque_limit/1 -> u_torque/1, Dot Product/2
  K_omega/1 -> torque_limit/1
  omega/1 -> Sum/2, sum_euler_x_omega/2  "omega"
  Sum2/1 -> sum_euler_x_omega/1, Unit Delay/1  "sum_euler_x_omega"
  Unit Delay/1 -> Sum2/2
  Dot Product/1 -> Sum2/1
  SectorSearch/1 -> Scope/1, a_e/1

== system starmac_system_embedded_test/robo_stix/lead_motor ==
  thrust_in : Inport  DataType=single  OutDataTypeStr=single
  Sum : Sum  Inputs=++-  AccumDataTypeStr=single  OutDataType=sfix(16)  OutScaling=2^0
  Unit Delay : UnitDelay  SampleTime=-1
  Unit Delay1 : UnitDelay  Orientation=left  SampleTime=-1
  a_1 : Gain  Orientation=up  Gain=4.3213919e-2  ParameterDataType=sfix(16)  ParameterScaling=2^0  OutDataTypeMode=single  OutDataType=sfix(16)  OutScaling=2^0  OutDataTypeStr=single
  b_1 : Gain  Orientation=down  Gain=-4.5225897  ParameterDataType=sfix(16)  ParameterScaling=2^0  OutDataTypeMode=single  OutDataType=sfix(16)  OutScaling=2^0  OutDataTypeStr=single
  b_2 : Gain  Orientation=down  Gain=5.4793758  ParameterDataType=sfix(16)  ParameterScaling=2^0  OutDataTypeMode=single  OutDataType=sfix(16)  OutScaling=2^0  OutDataTypeStr=single
  thrust_out : Outport  DataType=single  OutDataTypeStr=single
  wires:
  thrust_in/1 -> Unit Delay/1, b_2/1  "x"
  Unit Delay/1 -> b_1/1  "x_1"
  b_1/1 -> Sum/1
  b_2/1 -> Sum/2
  Sum/1 -> thrust_out/1, Unit Delay1/1  "y"
  a_1/1 -> Sum/3
  Unit Delay1/1 -> a_1/1  "y_1"

== system starmac_system_embedded_test/robo_stix/sensor_convert ==
  euler_s : Inport
  Ab_s : Inport  Port=2
  omega_s : Inport  Port=3
  accel_per_count : Gain  Gain=(9.81*7000)/(1e3*32768)  ParameterDataType=sfix(16)  ParameterScaling=2^0  OutDataTypeMode=single  OutDataType=sfix(16)  OutScaling=2^0  OutDataTypeStr=single
  radian_p_sec_per_count : Gain  Gain=8500/(1e3*32768)  ParameterDataType=sfix(16)  ParameterScaling=2^0  OutDataTypeMode=single  OutDataType=sfix(16)  OutScaling=2^0  OutDataTypeStr=single
  radian_per_count : Gain  Gain=pi/32768  ParameterDataType=sfix(16)  ParameterScaling=2^0  OutDataTypeMode=single  OutDataType=sfix(16)  OutScaling=2^0  OutDataTypeStr=single
  euler : Outport
  Ab : Outport  Port=2
  omega : Outport  Port=3
  wires:
  euler_s/1 -> radian_per_count/1
  radian_per_count/1 -> euler/1
  Ab_s/1 -> accel_per_count/1
  accel_per_count/1 -> Ab/1
  omega_s/1 -> radian_p_sec_per_count/1
  radian_p_sec_per_count/1 -> omega/1

== system starmac_system_embedded_test/robo_stix/u_T_u_torque_motor_thrust ==
  u_torque : Inport
  u_T : Inport  Port=2
  Mi : Gain  Gain=[0,1.6404,-.5319,.25;-1.6404,0,.5319,.25;0,-1.6404,-.5319,.25;1.6404,0,.5319,.25]  Multiplication=Matrix(K*u)  ParameterDataTypeMode=single  ParameterDataType=sfix(16)  ParameterScaling=2^0  ParamDataTypeStr=single  OutDataTypeMode=single  OutDataType=sfix(16)  OutScaling=2^0  OutDataTypeStr=single
  u_torque_u_T_mux : Stateflow chart
  cont_motor_thrust : Outport
  wires:
  u_torque/1 -> u_torque_u_T_mux/1(u_torque)
  u_T/1 -> u_torque_u_T_mux/2(u_T)
  Mi/1 -> cont_motor_thrust/1
  u_torque_u_T_mux/1(u_torque_u_T) -> Mi/1

== system starmac_system_embedded_test/sector_analysis/passive_filt ==
  In1 : Inport  Orientation=left
  Demux : Demux  Orientation=left  Outputs=[1 1 1]
  Mux : Mux  Orientation=left  Inputs=[1 1 1]
  Transfer Fcn : TransferFcn  Orientation=left  Numerator=[omega_n^2]  Denominator=[1 2*zeta*omega_n omega_n^2]
  Transfer Fcn1 : TransferFcn  Orientation=left  Numerator=[omega_n^2]  Denominator=[1 2*zeta*omega_n omega_n^2]
  Transfer Fcn2 : TransferFcn  Orientation=left  Numerator=[omega_n^2]  Denominator=[1 2*zeta*omega_n omega_n^2]
  Out1 : Outport  Orientation=left
  wires:
  Mux/1 -> Out1/1
  Transfer Fcn/1 -> Mux/1
  Transfer Fcn1/1 -> Mux/2
  Transfer Fcn2/1 -> Mux/3
  Demux/1 -> Transfer Fcn/1
  Demux/2 -> Transfer Fcn1/1
  Demux/3 -> Transfer Fcn2/1
  In1/1 -> Demux/1

== system starmac_system_embedded_test/sector_analysis/passive_filt1 ==
  In1 : Inport  Orientation=left
  Demux : Demux  Orientation=left  Outputs=[1 1 1]
  Mux : Mux  Orientation=left  Inputs=[1 1 1]
  Transfer Fcn : TransferFcn  Orientation=left  Numerator=[omega_n^2]  Denominator=[1 2*zeta*omega_n omega_n^2]
  Transfer Fcn1 : TransferFcn  Orientation=left  Numerator=[omega_n^2]  Denominator=[1 2*zeta*omega_n omega_n^2]
  Transfer Fcn2 : TransferFcn  Orientation=left  Numerator=[omega_n^2]  Denominator=[1 2*zeta*omega_n omega_n^2]
  Out1 : Outport  Orientation=left
  wires:
  In1/1 -> Demux/1
  Demux/3 -> Transfer Fcn2/1
  Demux/2 -> Transfer Fcn1/1
  Demux/1 -> Transfer Fcn/1
  Transfer Fcn2/1 -> Mux/3
  Transfer Fcn1/1 -> Mux/2
  Transfer Fcn/1 -> Mux/1
  Mux/1 -> Out1/1

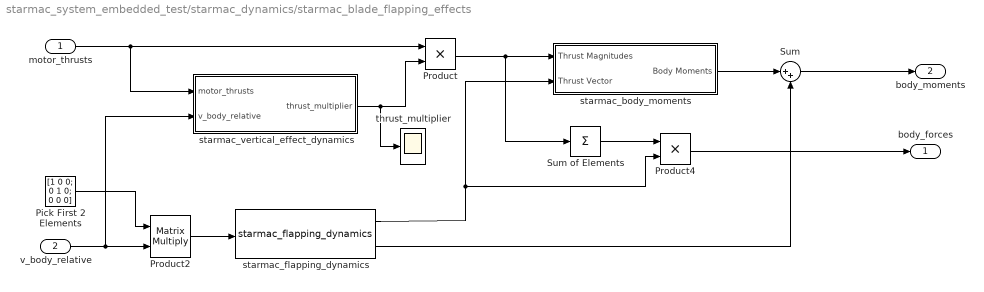
== system starmac_system_embedded_test/starmac_dynamics/starmac_blade_flapping_effects ==
  motor_thrusts : Inport  OutDataType=sfix(16)  OutScaling=2^0
  v_body_relative : Inport  Port=2  OutDataType=sfix(16)  OutScaling=2^0
  Pick First 2 Elements : Constant  Value=[1 0 0; 0 1 0; 0 0 0]  OutDataType=sfix(16)  OutScaling=2^0
  Product : Product  OutDataType=sfix(16)  OutScaling=2^0  RndMeth=Zero
  Product2 : Product  Multiplication=Matrix(*)  OutDataType=sfix(16)  OutScaling=2^0  RndMeth=Zero
  Product4 : Product  OutDataType=sfix(16)  OutScaling=2^0  RndMeth=Zero
  Sum : Sum  Inputs=|++  OutDataType=sfix(16)  OutScaling=2^0
  Sum of Elements : Sum  Inputs=+  OutDataType=sfix(16)  OutScaling=2^-10
  starmac_body_moments : Subsystem  AncestorBlock=aero_sim_lib/starmac_body_moments  mask{dx=.3048, dz=.07, K_torque=.47}
  starmac_flapping_dynamics : aero_sim_lib/starmac_flapping_dynamics  SystemSampleTime=-1  K_a1s=.009  K_beta=.23
  starmac_vertical_effect_dynamics : Subsystem  AncestorBlock=aero_sim_lib/starmac_vertical_effect_dynamics  mask{tau_motor=tau_motor, R=0.127, Alpha=(pi/180)*[-85:5:85], Vinf=[0:0.5:6], Thrust=9.8*[0.3:0.02:0.8]}
      mask prompts: tau_motor "motor time constant (s)"; R "radius of propeller (m)"; Alpha "Alpha (radians)"; Vinf "Vinf (radians)"; Thrust "Propeller Thrust (N)"
      mask init:
      | rho = 1.2;
      | A = pi*R^2;
      | Vh = sqrt(Thrust/(2*rho*A));
      | for i = 1:length(Vh)
      |     for j = 1:length(Vinf)
      |         for k = 1:length(Alpha)
      |             Vi(k,j,i) = find_vi(Vh(i),Vinf(j),Alpha(k));
      |             ToverTh(k,j,i) = min(10,max(0.1,Vh(i)/(Vi(k,j,i)+Vinf(j)*sin(Alpha(k)))));
      |         end
      |     end
      | end
  thrust_multiplier : Scope
      settings: YMin=0  YMax=1.5  SaveName=ScopeData7  Decimation=2
  body_forces : Outport  OutDataType=sfix(16)  OutScaling=2^0
  body_moments : Outport  Port=2  OutDataType=sfix(16)  OutScaling=2^0
  wires:
  starmac_flapping_dynamics/2 -> Sum/2
  Sum/1 -> body_moments/1
  starmac_body_moments/1(Body Moments) -> Sum/1
  starmac_flapping_dynamics/1 -> Product4/2, starmac_body_moments/2(Thrust Vector)
  Product4/1 -> body_forces/1
  Sum of Elements/1 -> Product4/1
  Product2/1 -> starmac_flapping_dynamics/1
  v_body_relative/1 -> Product2/2, starmac_vertical_effect_dynamics/2(v_body_relative)
  Pick First 2 Elements/1 -> Product2/1
  motor_thrusts/1 -> Product/1, starmac_vertical_effect_dynamics/1(motor_thrusts)
  starmac_vertical_effect_dynamics/1(thrust_multiplier) -> Product/2, thrust_multiplier/1
  Product/1 -> Sum of Elements/1, starmac_body_moments/1(Thrust Magnitudes)

== system starmac_system_embedded_test/gum_stix/body_to_inertial/inertial_vel_and pos_est ==
  Ab : Inport
  DT_integrator : Subsystem
  DT_integrator1 : Subsystem
  Vb : Outport
  Xb : Outport  Port=2
  wires:
  DT_integrator1/1(Xb) -> Xb/1
  Ab/1 -> DT_integrator/1(Ab)
  DT_integrator/1(Vb) -> Vb/1, DT_integrator1/1(Vb)

== system starmac_system_embedded_test/gum_stix/inertial_pos_controller/input_filter ==
  yaw_set : Inport  OutDataType=sfix(16)  OutScaling=2^0
  LinDiscSS1 : control_design_lib/LinDiscSS  SystemSampleTime=-1  Add=Add  Bdd=Bdd  Cdd=Cdd  Ddd=Ddd  x0=[0 0]  Tsamp=Tsamp
  yaw_r : Outport  OutDataType=sfix(16)  OutScaling=2^0
  wires:
  yaw_set/1 -> LinDiscSS1/1
  LinDiscSS1/1 -> yaw_r/1

== system starmac_system_embedded_test/gum_stix/inertial_pos_controller/vel_est ==
  Xe_set : Inport
  Sum : Sum  Inputs=++-  AccumDataTypeStr=single  OutDataType=sfix(16)  OutScaling=2^0
  Unit Delay : UnitDelay  SampleTime=-1
  Unit Delay1 : UnitDelay  Orientation=left  SampleTime=-1
  a_1 : Gain  Orientation=up  Gain=4.3213919e-002  ParameterDataType=sfix(16)  ParameterScaling=2^0  OutDataTypeMode=single  OutDataType=sfix(16)  OutScaling=2^0  OutDataTypeStr=single
  b_1 : Gain  Orientation=down  Gain=-4.7839306e+001  ParameterDataType=sfix(16)  ParameterScaling=2^0  OutDataTypeMode=single  OutDataType=sfix(16)  OutScaling=2^0  OutDataTypeStr=single
  b_2 : Gain  Orientation=down  Gain=4.7839306e+001  ParameterDataType=sfix(16)  ParameterScaling=2^0  OutDataTypeMode=single  OutDataType=sfix(16)  OutScaling=2^0  OutDataTypeStr=single
  Ve_set : Outport
  wires:
  Xe_set/1 -> Unit Delay/1, b_2/1  "x"
  Unit Delay/1 -> b_1/1  "x_1"
  b_1/1 -> Sum/1
  b_2/1 -> Sum/2
  Sum/1 -> Unit Delay1/1, Ve_set/1  "y"
  a_1/1 -> Sum/3
  Unit Delay1/1 -> a_1/1  "y_1"

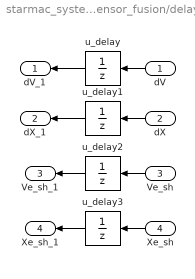
== system starmac_system_embedded_test/gum_stix/sensor_fusion/delays ==
  dV : Inport  Orientation=left
  dX : Inport  Orientation=left  Port=2
  Ve_sh : Inport  Orientation=left  Port=3
  Xe_sh : Inport  Orientation=left  Port=4
  u_delay{,1..3} (4 alike) : UnitDelay  Orientation=left  SampleTime=-1
  dV_1 : Outport  Orientation=left
  dX_1 : Outport  Orientation=left  Port=2
  Ve_sh_1 : Outport  Orientation=left  Port=3
  Xe_sh_1 : Outport  Orientation=left  Port=4
  wires:
  dV/1 -> u_delay/1
  u_delay/1 -> dV_1/1
  dX/1 -> u_delay1/1
  u_delay1/1 -> dX_1/1
  Ve_sh/1 -> u_delay2/1
  u_delay2/1 -> Ve_sh_1/1
  Xe_sh/1 -> u_delay3/1
  u_delay3/1 -> Xe_sh_1/1

== system starmac_system_embedded_test/gum_stix/sensor_fusion/if_end ==
  Xe_s : Inport
  Xe_f : Inport  Port=2
  dX_1p : Inport  Port=3
  Xe_sh_1p : Inport  Port=4
  If : If  NumInputs=2  IfExpression=(u1(1) ~= u2(1)) | (u1(2) ~= u2(2)) | (u1(3) ~= u2(3))
  If Action Subsystem : Subsystem  TreatAsAtomicUnit=on
  If Action Subsystem1 : Subsystem  TreatAsAtomicUnit=on
  Sum : Sum  Inputs=|++  OutDataTypeMode=single  OutDataType=sfix(16)  OutScaling=2^0  OutDataTypeStr=single
  Sum1 : Sum  Inputs=|++  OutDataTypeMode=single  OutDataType=sfix(16)  OutScaling=2^0  OutDataTypeStr=single
  Xe_sh_1 : Outport
  dX_1 : Outport  Port=2
  wires:
  If/1 -> If Action Subsystem/Action
  If/2 -> If Action Subsystem1/Action
  Xe_s/1 -> If Action Subsystem/1(Xe_s), If/1
  Xe_sh_1p/1 -> If/2, If Action Subsystem1/1(Xe_sh_1p)
  If Action Subsystem/1(Xe_sh_1) -> Sum/1
  If Action Subsystem/2(dX_1) -> Sum1/1
  If Action Subsystem1/1(Xe_sh_1) -> Sum/2
  If Action Subsystem1/2(dX_1) -> Sum1/2
  Sum/1 -> Xe_sh_1/1
  Xe_f/1 -> If Action Subsystem/2(Xe_f)
  Sum1/1 -> dX_1/1
  dX_1p/1 -> If Action Subsystem1/2(dX_1p)

== system starmac_system_embedded_test/gum_stix/sensor_fusion/if_end1 ==
  Ve_s : Inport
  Ve_f : Inport  Port=2
  dV_1p : Inport  Port=3
  Ve_sh_1p : Inport  Port=4
  If : If  NumInputs=2  IfExpression=(u1(1) ~= u2(1)) | (u1(2) ~= u2(2)) | (u1(3) ~= u2(3))
  If Action Subsystem : Subsystem  TreatAsAtomicUnit=on
  If Action Subsystem1 : Subsystem  TreatAsAtomicUnit=on
  Sum : Sum  Inputs=|++  OutDataTypeMode=single  OutDataType=sfix(16)  OutScaling=2^0  OutDataTypeStr=single
  Sum1 : Sum  Inputs=|++  OutDataTypeMode=single  OutDataType=sfix(16)  OutScaling=2^0  OutDataTypeStr=single
  Ve_sh_1 : Outport
  dV_1 : Outport  Port=2
  wires:
  dV_1p/1 -> If Action Subsystem1/2(dV_1p)
  Sum1/1 -> dV_1/1
  Ve_f/1 -> If Action Subsystem/2(Ve_f)
  Sum/1 -> Ve_sh_1/1
  If Action Subsystem1/2(dV_1) -> Sum1/2
  If Action Subsystem1/1(Ve_sh_1) -> Sum/2
  If Action Subsystem/2(dV_1) -> Sum1/1
  If Action Subsystem/1(Ve_sh_1) -> Sum/1
  Ve_sh_1p/1 -> If Action Subsystem1/1(Ve_sh_1p), If/2
  Ve_s/1 -> If/1, If Action Subsystem/1(Ve_s)
  If/2 -> If Action Subsystem1/Action
  If/1 -> If Action Subsystem/Action

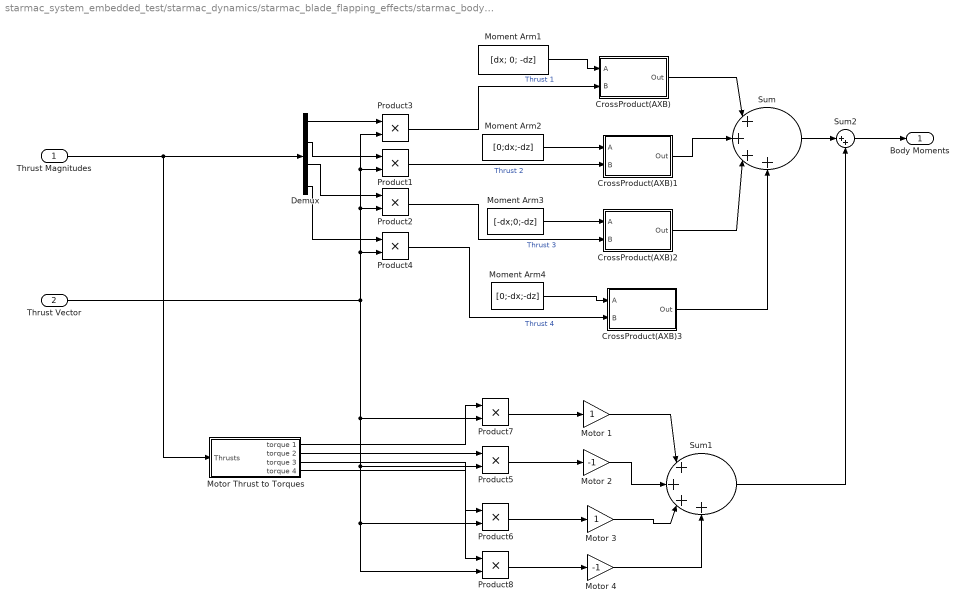
== system starmac_system_embedded_test/starmac_dynamics/starmac_blade_flapping_effects/starmac_body_moments ==
  Thrust Magnitudes : Inport  OutDataType=sfix(16)  OutScaling=2^0
  Thrust Vector : Inport  Port=2  OutDataType=sfix(16)  OutScaling=2^0
  CrossProduct(AXB) : Subsystem
  CrossProduct(AXB)1 : Subsystem
  CrossProduct(AXB)2 : Subsystem
  CrossProduct(AXB)3 : Subsystem
  Demux : Demux
  Moment Arm1 : Constant  Value=[dx; 0; -dz]  OutDataType=sfix(16)  OutScaling=2^0
  Moment Arm2 : Constant  Value=[0;dx;-dz]  OutDataType=sfix(16)  OutScaling=2^0
  Moment Arm3 : Constant  Value=[-dx;0;-dz]  OutDataType=sfix(16)  OutScaling=2^0
  Moment Arm4 : Constant  Value=[0;-dx;-dz]  OutDataType=sfix(16)  OutScaling=2^0
  Motor 1 : Gain  ParameterDataType=sfix(16)  ParameterScaling=2^0  OutDataType=sfix(16)  OutScaling=2^0
  Motor 2 : Gain  Gain=-1  ParameterDataType=sfix(16)  ParameterScaling=2^0  OutDataType=sfix(16)  OutScaling=2^0
  Motor 3 : Gain  ParameterDataType=sfix(16)  ParameterScaling=2^0  OutDataType=sfix(16)  OutScaling=2^0
  Motor 4 : Gain  Gain=-1  ParameterDataType=sfix(16)  ParameterScaling=2^0  OutDataType=sfix(16)  OutScaling=2^0
  Motor Thrust to Torques : Subsystem
  Product{1..8} (8 alike) : Product  OutDataType=sfix(16)  OutScaling=2^0  RndMeth=Zero
  Sum : Sum  Inputs=|++++  OutDataType=sfix(16)  OutScaling=2^0
  Sum1 : Sum  Inputs=|++++  OutDataType=sfix(16)  OutScaling=2^0
  Sum2 : Sum  Inputs=|++  OutDataType=sfix(16)  OutScaling=2^0
  Body Moments : Outport  OutDataType=sfix(16)  OutScaling=2^0
  wires:
  CrossProduct(AXB)1/1(Out) -> Sum/2
  Motor Thrust to Torques/4(torque 4) -> Product8/1
  Motor Thrust to Torques/3(torque 3) -> Product6/1
  Motor Thrust to Torques/2(torque 2) -> Product5/1
  Motor Thrust to Torques/1(torque 1) -> Product7/1
  Product8/1 -> Motor 4/1
  Product6/1 -> Motor 3/1
  Product5/1 -> Motor 2/1
  Product7/1 -> Motor 1/1
  Sum2/1 -> Body Moments/1
  Sum1/1 -> Sum2/2
  Sum/1 -> Sum2/1
  Motor 4/1 -> Sum1/4
  Motor 3/1 -> Sum1/3
  Motor 2/1 -> Sum1/2
  Motor 1/1 -> Sum1/1
  CrossProduct(AXB)3/1(Out) -> Sum/4
  CrossProduct(AXB)2/1(Out) -> Sum/3
  CrossProduct(AXB)/1(Out) -> Sum/1
  Product4/1 -> CrossProduct(AXB)3/2(B)  "Thrust 4"
  Moment Arm4/1 -> CrossProduct(AXB)3/1(A)
  Product2/1 -> CrossProduct(AXB)2/2(B)  "Thrust 3"
  Moment Arm3/1 -> CrossProduct(AXB)2/1(A)
  Product1/1 -> CrossProduct(AXB)1/2(B)  "Thrust 2"
  Moment Arm2/1 -> CrossProduct(AXB)1/1(A)
  Product3/1 -> CrossProduct(AXB)/2(B)  "Thrust 1"
  Moment Arm1/1 -> CrossProduct(AXB)/1(A)
  Thrust Vector/1 -> Product8/2, Product6/2, Product5/2, Product7/2, Product4/2, Product2/2, Product1/2, Product3/2
  Demux/4 -> Product4/1
  Demux/3 -> Product2/1
  Demux/2 -> Product1/1
  Demux/1 -> Product3/1
  Thrust Magnitudes/1 -> Motor Thrust to Torques/1(Thrusts), Demux/1

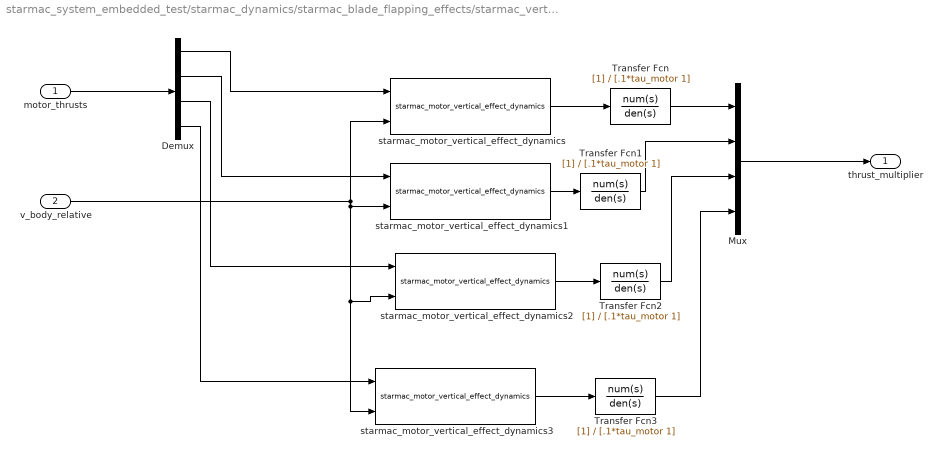
== system starmac_system_embedded_test/starmac_dynamics/starmac_blade_flapping_effects/starmac_vertical_effect_dynamics ==
  motor_thrusts : Inport  OutDataType=sfix(16)  OutScaling=2^0
  v_body_relative : Inport  Port=2  OutDataType=sfix(16)  OutScaling=2^0
  Demux : Demux
  Mux : Mux
  Transfer Fcn{,1..3} (4 alike) : TransferFcn  Denominator=[.1*tau_motor 1]
  starmac_motor_vertical_effect_dynamics{,1..3} (4 alike) : aero_sim_lib/starmac_motor_vertical_effect_dynamics  SystemSampleTime=-1  tau_motor=tau_motor  R=R  Alpha=Alpha  Vinf=Vinf  Vh=Vh  ToverTh=ToverTh
  thrust_multiplier : Outport  OutDataType=sfix(16)  OutScaling=2^0
  wires:
  motor_thrusts/1 -> Demux/1
  Mux/1 -> thrust_multiplier/1
  Demux/1 -> starmac_motor_vertical_effect_dynamics/1
  Demux/2 -> starmac_motor_vertical_effect_dynamics1/1
  Demux/3 -> starmac_motor_vertical_effect_dynamics2/1
  Demux/4 -> starmac_motor_vertical_effect_dynamics3/1
  starmac_motor_vertical_effect_dynamics/1 -> Transfer Fcn/1
  starmac_motor_vertical_effect_dynamics1/1 -> Transfer Fcn1/1
  starmac_motor_vertical_effect_dynamics2/1 -> Transfer Fcn2/1
  starmac_motor_vertical_effect_dynamics3/1 -> Transfer Fcn3/1
  v_body_relative/1 -> starmac_motor_vertical_effect_dynamics2/2, starmac_motor_vertical_effect_dynamics3/2, starmac_motor_vertical_effect_dynamics1/2, starmac_motor_vertical_effect_dynamics/2
  Transfer Fcn/1 -> Mux/1
  Transfer Fcn1/1 -> Mux/2
  Transfer Fcn2/1 -> Mux/3
  Transfer Fcn3/1 -> Mux/4

== system starmac_system_embedded_test/gum_stix/body_to_inertial/inertial_vel_and pos_est/DT_integrator ==
  Ab : Inport
  Sum : Sum  Inputs=++|  OutDataTypeMode=single  OutDataType=sfix(16)  OutScaling=2^0  OutDataTypeStr=single
  Sum1 : Sum  Inputs=|++  AccumDataTypeStr=single  OutDataType=sfix(16)  OutScaling=2^0
  negate : Gain  Gain=.5*.02  ParameterDataType=sfix(16)  ParameterScaling=2^0  OutDataTypeMode=single  OutDataType=sfix(16)  OutScaling=2^0  OutDataTypeStr=single
  u_delay : UnitDelay  SampleTime=-1
  u_delay1 : UnitDelay  Orientation=left  SampleTime=-1
  Vb : Outport
  wires:
  Ab/1 -> u_delay/1, Sum/2
  u_delay/1 -> Sum/1
  Sum/1 -> negate/1
  negate/1 -> Sum1/1
  Sum1/1 -> u_delay1/1, Vb/1
  u_delay1/1 -> Sum1/2

== system starmac_system_embedded_test/gum_stix/body_to_inertial/inertial_vel_and pos_est/DT_integrator1 ==
  Vb : Inport
  Sum : Sum  Inputs=++|  OutDataTypeMode=single  OutDataType=sfix(16)  OutScaling=2^0  OutDataTypeStr=single
  Sum1 : Sum  Inputs=|++  OutDataTypeMode=single  OutDataType=sfix(16)  OutScaling=2^0  OutDataTypeStr=single
  negate : Gain  Gain=.5*.02  ParameterDataType=sfix(16)  ParameterScaling=2^0  OutDataTypeMode=single  OutDataType=sfix(16)  OutScaling=2^0  OutDataTypeStr=single
  u_delay : UnitDelay  SampleTime=-1
  u_delay1 : UnitDelay  Orientation=left  SampleTime=-1
  Xb : Outport  PortDimensions=[3]  DataType=single  OutDataTypeStr=single
  wires:
  u_delay1/1 -> Sum1/2
  Sum1/1 -> Xb/1, u_delay1/1
  negate/1 -> Sum1/1
  Sum/1 -> negate/1
  u_delay/1 -> Sum/1
  Vb/1 -> Sum/2, u_delay/1

== system starmac_system_embedded_test/gum_stix/sensor_fusion/if_end/If Action Subsystem ==
  Xe_s : Inport  OutDataType=sfix(16)  OutScaling=2^0
  Xe_f : Inport  Port=2  OutDataType=sfix(16)  OutScaling=2^0
  Action Port : ActionPort  InitializeStates=reset  ActionType=then
  Sum : Sum  Inputs=-+|  OutDataTypeMode=single  OutDataType=sfix(16)  OutScaling=2^0  OutDataTypeStr=single
  Xe_sh_1 : Outport  OutDataType=sfix(16)  OutScaling=2^0  OutputWhenDisabled=reset  InitialOutput=zeros(1,3,'single')
  dX_1 : Outport  Port=2  OutDataType=sfix(16)  OutScaling=2^0  OutputWhenDisabled=reset  InitialOutput=zeros(1,3,'single')
  wires:
  Xe_s/1 -> Xe_sh_1/1, Sum/1
  Xe_f/1 -> Sum/2
  Sum/1 -> dX_1/1

== system starmac_system_embedded_test/gum_stix/sensor_fusion/if_end/If Action Subsystem1 ==
  Xe_sh_1p : Inport  OutDataType=sfix(16)  OutScaling=2^0
  dX_1p : Inport  Port=2  OutDataType=sfix(16)  OutScaling=2^0
  Action Port : ActionPort  InitializeStates=reset  ActionType=else
  Xe_sh_1 : Outport  DataType=single  OutDataType=sfix(16)  OutScaling=2^0  OutDataTypeStr=single  OutputWhenDisabled=reset  InitialOutput=zeros(1,3,'single')
  dX_1 : Outport  Port=2  DataType=single  OutDataType=sfix(16)  OutScaling=2^0  OutDataTypeStr=single  OutputWhenDisabled=reset  InitialOutput=zeros(1,3,'single')
  wires:
  dX_1p/1 -> dX_1/1
  Xe_sh_1p/1 -> Xe_sh_1/1

== system starmac_system_embedded_test/gum_stix/sensor_fusion/if_end1/If Action Subsystem ==
  Ve_s : Inport  OutDataType=sfix(16)  OutScaling=2^0
  Ve_f : Inport  Port=2  OutDataType=sfix(16)  OutScaling=2^0
  Action Port : ActionPort  InitializeStates=reset  ActionType=then
  Sum : Sum  Inputs=-+|  OutDataTypeMode=single  OutDataType=sfix(16)  OutScaling=2^0  OutDataTypeStr=single
  Ve_sh_1 : Outport  OutDataType=sfix(16)  OutScaling=2^0  OutputWhenDisabled=reset  InitialOutput=zeros(1,3,'single')
  dV_1 : Outport  Port=2  OutDataType=sfix(16)  OutScaling=2^0  OutputWhenDisabled=reset  InitialOutput=zeros(1,3,'single')
  wires:
  Sum/1 -> dV_1/1
  Ve_f/1 -> Sum/2
  Ve_s/1 -> Sum/1, Ve_sh_1/1

== system starmac_system_embedded_test/gum_stix/sensor_fusion/if_end1/If Action Subsystem1 ==
  Ve_sh_1p : Inport  OutDataType=sfix(16)  OutScaling=2^0
  dV_1p : Inport  Port=2  OutDataType=sfix(16)  OutScaling=2^0
  Action Port : ActionPort  InitializeStates=reset  ActionType=else
  Ve_sh_1 : Outport  DataType=single  OutDataType=sfix(16)  OutScaling=2^0  OutDataTypeStr=single  OutputWhenDisabled=reset  InitialOutput=zeros(1,3,'single')
  dV_1 : Outport  Port=2  DataType=single  OutDataType=sfix(16)  OutScaling=2^0  OutDataTypeStr=single  OutputWhenDisabled=reset  InitialOutput=zeros(1,3,'single')
  wires:
  Ve_sh_1p/1 -> Ve_sh_1/1
  dV_1p/1 -> dV_1/1

== system starmac_system_embedded_test/starmac_dynamics/starmac_blade_flapping_effects/starmac_body_moments/CrossProduct(AXB) ==
  A : Inport  OutDataType=sfix(16)  OutScaling=2^0
  B : Inport  Port=2  OutDataType=sfix(16)  OutScaling=2^0
  Fcn : Fcn  Expr=u[2]*u[6]-u[3]*u[5]
  Fcn1 : Fcn  Expr=u[3]*u[4]-u[1]*u[6]
  Fcn2 : Fcn  Expr=u[1]*u[5]-u[2]*u[4]
  Mux : Mux  Inputs=2
  Mux1 : Mux  Inputs=3
  Out : Outport  OutDataType=sfix(16)  OutScaling=2^0
  wires:
  Mux1/1 -> Out/1
  Fcn2/1 -> Mux1/3
  Fcn1/1 -> Mux1/2
  Fcn/1 -> Mux1/1
  Mux/1 -> Fcn2/1, Fcn1/1, Fcn/1
  B/1 -> Mux/2
  A/1 -> Mux/1

== system starmac_system_embedded_test/starmac_dynamics/starmac_blade_flapping_effects/starmac_body_moments/CrossProduct(AXB)1 ==
  A : Inport  OutDataType=sfix(16)  OutScaling=2^0
  B : Inport  Port=2  OutDataType=sfix(16)  OutScaling=2^0
  Fcn : Fcn  Expr=u[2]*u[6]-u[3]*u[5]
  Fcn1 : Fcn  Expr=u[3]*u[4]-u[1]*u[6]
  Fcn2 : Fcn  Expr=u[1]*u[5]-u[2]*u[4]
  Mux : Mux  Inputs=2
  Mux1 : Mux  Inputs=3
  Out : Outport  OutDataType=sfix(16)  OutScaling=2^0
  wires:
  A/1 -> Mux/1
  B/1 -> Mux/2
  Mux/1 -> Fcn/1, Fcn1/1, Fcn2/1
  Fcn/1 -> Mux1/1
  Fcn1/1 -> Mux1/2
  Fcn2/1 -> Mux1/3
  Mux1/1 -> Out/1

== system starmac_system_embedded_test/starmac_dynamics/starmac_blade_flapping_effects/starmac_body_moments/CrossProduct(AXB)2 ==
  A : Inport  OutDataType=sfix(16)  OutScaling=2^0
  B : Inport  Port=2  OutDataType=sfix(16)  OutScaling=2^0
  Fcn : Fcn  Expr=u[2]*u[6]-u[3]*u[5]
  Fcn1 : Fcn  Expr=u[3]*u[4]-u[1]*u[6]
  Fcn2 : Fcn  Expr=u[1]*u[5]-u[2]*u[4]
  Mux : Mux  Inputs=2
  Mux1 : Mux  Inputs=3
  Out : Outport  OutDataType=sfix(16)  OutScaling=2^0
  wires:
  Mux1/1 -> Out/1
  Fcn2/1 -> Mux1/3
  Fcn1/1 -> Mux1/2
  Fcn/1 -> Mux1/1
  Mux/1 -> Fcn2/1, Fcn1/1, Fcn/1
  B/1 -> Mux/2
  A/1 -> Mux/1
